simulink model "PUMAA"  (R2021a)
settings: Solver=VariableStepAuto  StartTime=0.0  StopTime=1451.7  RelTol=1e-3
undefined symbols (not defined in the file): sigbuilder_block, X, Y, Z
libraries: sm_lib x25, nesl_utility x15, pid_lib x6
settings Model: Creator=legen  LastModifiedBy=MSI

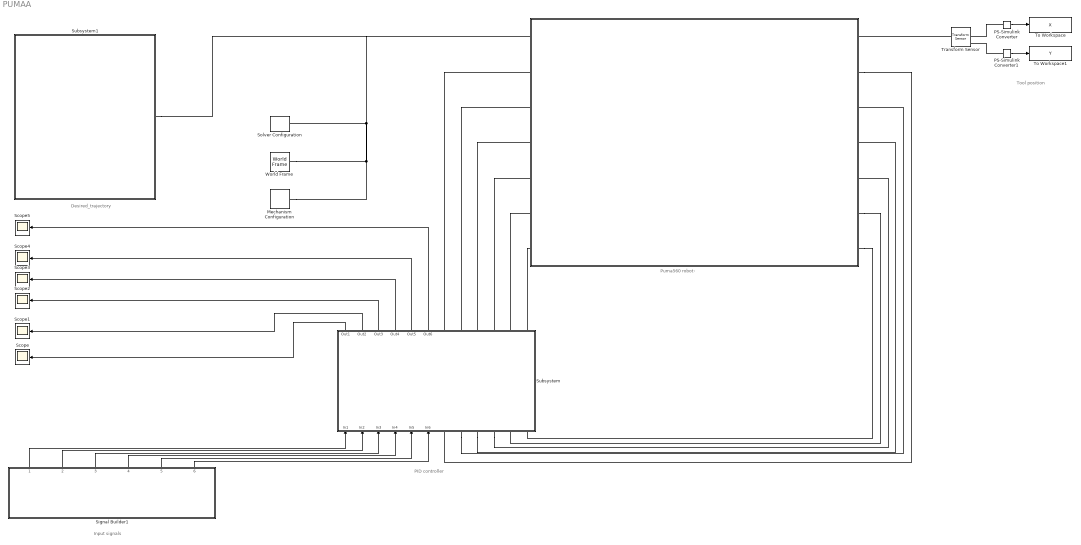
== system PUMAA ==
  note: Desired_trajectory
  note: Puma560 robot
  note: PID controller
  note: Input signals
  note: Tool position
  " ." : Subsystem
      mask Display: image('Puma.png'); % Use "Edit Image" on toolstrip to change.
  Mechanism Configuration : sm_lib/Utilities/Mechanism Configuration  UniformGravity=Constant  GravityVector=[0 0 -9.80665]  GravityVectorUnits=m/s^2  GravityUnits=m/s^2  LinearizationDelta=0.0001  JointModeTransitionNonlinearIterations=2
  PS-Simulink Converter : nesl_utility/PS-Simulink Converter  PhysicalDomain=network_engine_domain  SubClassName=ps_output  LeftPortType=input  RightPortType=output  PseudoPeriodic=off  Frequencies=[]  Unit=inherit  AffineConversion=off
      settings: SourceProductBaseCode=PW,SS
  PS-Simulink Converter1 : nesl_utility/PS-Simulink Converter  PhysicalDomain=network_engine_domain  SubClassName=ps_output  LeftPortType=input  RightPortType=output  PseudoPeriodic=off  Frequencies=[]  Unit=inherit  AffineConversion=off
      settings: SourceProductBaseCode=PW,SS
  Scope{,1..5} (6 alike) : Scope
  Signal Builder1 : Subsystem  Tag=STV Subsys  LoadFcn=sigbuilder_block('load');  StartFcn=sigbuilder_block('start');  StopFcn=sigbuilder_block('stop');  ClipboardFcn=sigbuilder_block('clipboard');  mask(Sigbuilder block){tuvar=[0:10]}
      mask help: Simulink:masks:SigbuilderBlock_MD
      mask init:
      | if ~strcmp(get_param(bdroot(gcbh),'SimulationStatus'),'stopped') tuvar = sigbuilder_block('maskInit'); end
      settings: CopyFcn=sigbuilder_block('copy');  DeleteFcn=sigbuilder_block('delete');  ModelCloseFcn=sigbuilder_block('modelClose');  PreSaveFcn=sigbuilder_block('preSave');  PauseFcn=sigbuilder_block('pause');  ContinueFcn=sigbuilder_block('continue');  NameChangeFcn=sigbuilder_block('namechange');  OpenFcn=sigbuilder_block('open',[437.6 153 550.4 359.25 ]);  CloseFcn=sigbuilder_block('close');
      mask Display: plot(0, 0, 100, 100,[2, 2, 32, 32, 2], [68, 8, 8, 68, 68],[32, 2], [38, 38], [32, 19, 2],[53, 60, 44], [32, 17, 17, 2],[16, 16, 31, 31]);txt = getActiveGroup(gcbh);text(2, 100, txt,'verticalAlignment', 'top');
  Solver Configuration : nesl_utility/Solver Configuration  PhysicalDomain=network_engine_domain  SubClassName=solver  LeftPortType=input  RightPortType=generic  Tones=[]  Harmonics=[]  SimulateNoise=off  Profile=off  UseLocalSampling=off  EnableSwitchedLinearOptims=on  FrequencyDomain=off  UseCCode=off  RelTol=0.001  AbsTol=1e-06  MinStep=1e-09  ToWorkspace=off  RevertToSquareIcSolve=off  NumHomotopyIterations=100  PhasorMode=off  PhasorModeNumHarmonics=1  DoDC=off  ResidualTolerance=1e-09  UseLocalSolver=off  LocalSolverChoice=NE_BACKWARD_EULER_ADVANCER  LocalSolverSampleTime=0.001  DoFixedCost=off  MaxNonlinIter=3  MaxModeIter=2  ComputeImpulses=off  ImpulseIterations=2  LinearAlgebra=Sparse  EquationFormulation=NE_TIME_EF  DelaysMemoryBudget=1024  AutomaticFiltering=on  FilteringTimeConstant=0.001  PartitionStorageMethod=AS_NEEDED  PartitionMemoryBudget=1024  PartitionMethod=FAST
      settings: SourceProductBaseCode=PW,SS
  Subsystem : Subsystem
      mask Display: image('PID-Controller-Explained.png'); % Use "Edit Image" on toolstrip to change.
  Subsystem1 : Subsystem
      mask Display: image('trajectory.png'); % Use "Edit Image" on toolstrip to change.
  To Workspace : ToWorkspace  VariableName=X  SampleTime=0.1
  To Workspace1 : ToWorkspace  VariableName=Y  SampleTime=0.1
  Transform Sensor : sm_lib/Frames and Transforms/Transform Sensor  MeasurementFrame=World  SenseAngle=off  SenseAxis=off  SenseAngle1=off  SenseAngle2=off  SenseAngle3=off  SenseQ=off  SenseR=off  SenseOmegaX=off  SenseOmegaY=off  SenseOmegaZ=off  SenseOmega1=off  SenseOmega2=off  SenseOmega3=off  SenseQDot=off  SenseRDot=off  SenseAlphaX=off  SenseAlphaY=off  SenseAlphaZ=off  SenseAlpha1=off  SenseAlpha2=off  SenseAlpha3=off  SenseQDDot=off  SenseRDDot=off  SenseX=on  SenseY=on  SenseZ=off  SenseRad=off  SenseAzim=off  SenseDist=off  SenseInc=off  SenseXDot=off  SenseYDot=off  SenseZDot=off  SenseRadDot=off  SenseAzimDot=off  SenseDistDot=off  SenseIncDot=off  SenseXDDot=off  SenseYDDot=off  SenseZDDot=off  SenseRadDDot=off  SenseAzimDDot=off  SenseDistDDot=off  SenseIncDDot=off
  World Frame : sm_lib/Frames and Transforms/World Frame
  wires:
  PS-Simulink Converter/1 -> To Workspace/1
  PS-Simulink Converter1/1 -> To Workspace1/1
  Signal Builder1/1(Imported_Signal 1) -> Subsystem/1(In1)
  Signal Builder1/2(Imported_Signal 2) -> Subsystem/2(In2)
  Signal Builder1/3(Imported_Signal 3) -> Subsystem/3(In3)
  Signal Builder1/4(Imported_Signal 4) -> Subsystem/4(In4)
  Signal Builder1/5(Imported_Signal 5) -> Subsystem/5(In5)
  Signal Builder1/6(Imported_Signal 6) -> Subsystem/6(In6)
  Subsystem/1(Out1) -> Scope/1
  Subsystem/2(Out2) -> Scope1/1
  Subsystem/3(Out3) -> Scope2/1
  Subsystem/4(Out4) -> Scope3/1
  Subsystem/5(Out5) -> Scope4/1
  Subsystem/6(Out6) -> Scope5/1
  connections:
  Mechanism Configuration/RConn1 -- Subsystem1/LConn1 -- " ."/LConn1 -- Solver Configuration/RConn1 -- World Frame/RConn1
  PS-Simulink Converter1/LConn1 -- Transform Sensor/RConn3
  PS-Simulink Converter/LConn1 -- Transform Sensor/RConn2
  Transform Sensor/LConn1 -- " ."/RConn1
  Subsystem/RConn1 -- " ."/LConn2
  " ."/RConn2 -- Subsystem/LConn1
  Subsystem/RConn2 -- " ."/LConn3
  Subsystem/LConn2 -- " ."/RConn3
  Subsystem/RConn3 -- " ."/LConn4
  Subsystem/LConn3 -- " ."/RConn4
  Subsystem/RConn4 -- " ."/LConn5
  Subsystem/LConn4 -- " ."/RConn5
  Subsystem/RConn5 -- " ."/LConn6
  " ."/RConn6 -- Subsystem/LConn5
  Subsystem/RConn6 -- " ."/LConn7
  " ."/RConn7 -- Subsystem/LConn6

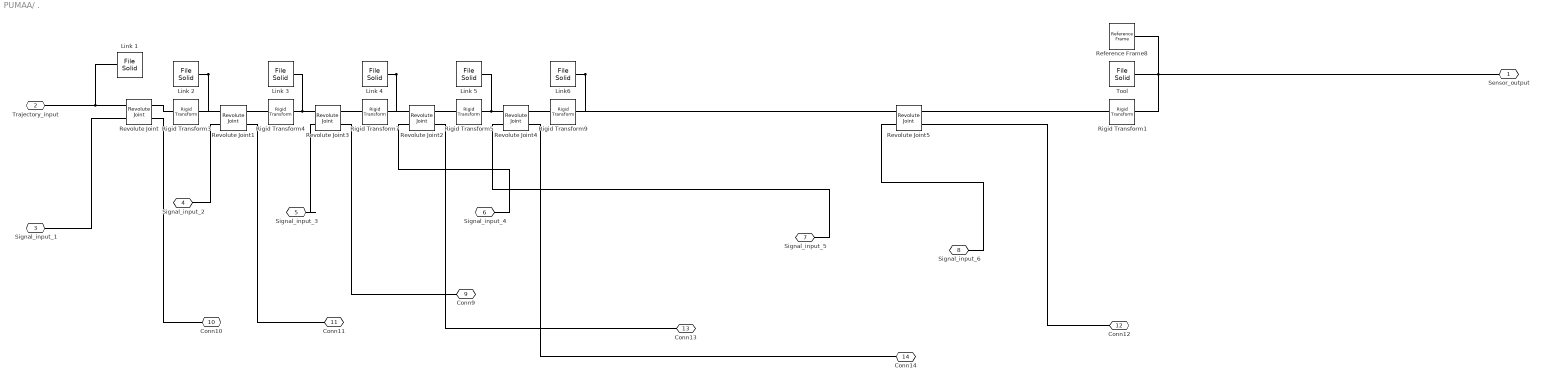
== system PUMAA/ . ==
  "Link 1 " : sm_lib/Body Elements/File Solid  ExtGeomFileName=C:\Users\MSI\Downloads\Robotics\Robotics\link0.stl  UnitType=Custom  ExtGeomFileUnits=m  StepReaderType=HEX  ExportConvexHullGeometry=off  InertiaType=Custom  Mass=0  MassUnits=kg  CenterOfMass=[0 0 0]  CenterOfMassUnits=m  MomentsOfInertia=[0 0.35 0]  MomentsOfInertiaUnits=kg*m^2  ProductsOfInertia=[0 0 0]  ProductsOfInertiaUnits=kg*m^2  BasedOnType=Mass  Density=1000  DensityUnits=kg/m^3  DoExposeReferenceFrame=on  SerializedFrames=<Frames/>  GraphicType=FromGeometry  MarkerShape=Sphere  MarkerSize=10  GraphicVisPropType=SimpleVisualProperties  GraphicDiffuseColor=[0.5 0.5 0.5]  GraphicSpecularColor=[0.5 0.5 0.5 1.0]  GraphicAmbientColor=[0.15 0.15 0.15 1.0]  GraphicEmissiveColor=[0.0 0.0 0.0 1.0]  GraphicShininess=75  GraphicOpacity=1.0
  Link 2 : sm_lib/Body Elements/File Solid  ExtGeomFileName=C:\Users\MSI\Downloads\Robotics\Robotics\link1.stl  UnitType=Custom  ExtGeomFileUnits=m  StepReaderType=HEX  ExportConvexHullGeometry=off  InertiaType=Custom  Mass=17.4  MassUnits=kg  CenterOfMass=[-0.3638 0.006 0.2275]  CenterOfMassUnits=m  MomentsOfInertia=[0.13 0.524 0.539]  MomentsOfInertiaUnits=kg*m^2  ProductsOfInertia=[0 0 0]  ProductsOfInertiaUnits=kg*m^2  BasedOnType=Density  Density=1000  DensityUnits=kg/m^3  DoExposeReferenceFrame=on  SerializedFrames=<Frames/>  GraphicType=FromGeometry  MarkerShape=Sphere  MarkerSize=10  GraphicVisPropType=SimpleVisualProperties  GraphicDiffuseColor=[0.5 0.5 0.5]  GraphicSpecularColor=[0.5 0.5 0.5 1.0]  GraphicAmbientColor=[0.15 0.15 0.15 1.0]  GraphicEmissiveColor=[0.0 0.0 0.0 1.0]  GraphicShininess=75  GraphicOpacity=1.0
  "Link 3 " : sm_lib/Body Elements/File Solid  ExtGeomFileName=C:\Users\MSI\Downloads\Robotics\Robotics\link2.stl  UnitType=Custom  ExtGeomFileUnits=m  StepReaderType=HEX  ExportConvexHullGeometry=off  InertiaType=Custom  Mass=4.8  MassUnits=kg  CenterOfMass="[-0.0203     -0.0141     0.07]"  CenterOfMassUnits=m  MomentsOfInertia=[0.066 0.086 0.0125]  MomentsOfInertiaUnits=kg*m^2  ProductsOfInertia=[0 0 0]  ProductsOfInertiaUnits=kg*m^2  BasedOnType=Density  Density=1000  DensityUnits=kg/m^3  DoExposeReferenceFrame=on  SerializedFrames=<Frames/>  GraphicType=FromGeometry  MarkerShape=Sphere  MarkerSize=10  GraphicVisPropType=SimpleVisualProperties  GraphicDiffuseColor=[0.5 0.5 0.5]  GraphicSpecularColor=[0.5 0.5 0.5 1.0]  GraphicAmbientColor=[0.15 0.15 0.15 1.0]  GraphicEmissiveColor=[0.0 0.0 0.0 1.0]  GraphicShininess=75  GraphicOpacity=1.0
  Link 4 : sm_lib/Body Elements/File Solid  ExtGeomFileName=C:\Users\MSI\Downloads\Robotics\Robotics\link3.stl  UnitType=Custom  ExtGeomFileUnits=m  StepReaderType=HEX  ExportConvexHullGeometry=off  InertiaType=Custom  Mass=0.82  MassUnits=kg  CenterOfMass="[0           0.019       0]"  CenterOfMassUnits=m  MomentsOfInertia=[0.0018 0.0013 0.0018]  MomentsOfInertiaUnits=kg*m^2  ProductsOfInertia=[0 0 0]  ProductsOfInertiaUnits=kg*m^2  BasedOnType=Density  Density=1000  DensityUnits=kg/m^3  DoExposeReferenceFrame=on  SerializedFrames=<Frames/>  GraphicType=FromGeometry  MarkerShape=Sphere  MarkerSize=10  GraphicVisPropType=SimpleVisualProperties  GraphicDiffuseColor=[0.5 0.5 0.5]  GraphicSpecularColor=[0.5 0.5 0.5 1.0]  GraphicAmbientColor=[0.15 0.15 0.15 1.0]  GraphicEmissiveColor=[0.0 0.0 0.0 1.0]  GraphicShininess=75  GraphicOpacity=1.0
  Link 5 : sm_lib/Body Elements/File Solid  ExtGeomFileName=C:\Users\MSI\Downloads\Robotics\Robotics\link4.stl  UnitType=Custom  ExtGeomFileUnits=m  StepReaderType=HEX  ExportConvexHullGeometry=off  InertiaType=Custom  Mass=0.34  MassUnits=kg  CenterOfMass=[0 0 0]  CenterOfMassUnits=m  MomentsOfInertia=[0.0003 0.0004 0.0003]  MomentsOfInertiaUnits=kg*m^2  ProductsOfInertia=[0 0 0]  ProductsOfInertiaUnits=kg*m^2  BasedOnType=Density  Density=1000  DensityUnits=kg/m^3  DoExposeReferenceFrame=on  SerializedFrames=<Frames/>  GraphicType=FromGeometry  MarkerShape=Sphere  MarkerSize=10  GraphicVisPropType=SimpleVisualProperties  GraphicDiffuseColor=[0.5 0.5 0.5]  GraphicSpecularColor=[0.5 0.5 0.5 1.0]  GraphicAmbientColor=[0.15 0.15 0.15 1.0]  GraphicEmissiveColor=[0.0 0.0 0.0 1.0]  GraphicShininess=75  GraphicOpacity=1.0
  Link6 : sm_lib/Body Elements/File Solid  ExtGeomFileName=C:\Users\MSI\Downloads\Robotics\Robotics\link5.stl  UnitType=Custom  ExtGeomFileUnits=m  StepReaderType=HEX  ExportConvexHullGeometry=off  InertiaType=Custom  Mass=0.09  MassUnits=kg  CenterOfMass=[0 0 0.032]  CenterOfMassUnits=m  MomentsOfInertia=[0.00015 0.00015 4e-5]  MomentsOfInertiaUnits=kg*m^2  ProductsOfInertia=[0 0 0]  ProductsOfInertiaUnits=kg*m^2  BasedOnType=Density  Density=1000  DensityUnits=kg/m^3  DoExposeReferenceFrame=on  SerializedFrames=<Frames/>  GraphicType=FromGeometry  MarkerShape=Sphere  MarkerSize=10  GraphicVisPropType=SimpleVisualProperties  GraphicDiffuseColor=[0.5 0.5 0.5]  GraphicSpecularColor=[0.5 0.5 0.5 1.0]  GraphicAmbientColor=[0.15 0.15 0.15 1.0]  GraphicEmissiveColor=[0.0 0.0 0.0 1.0]  GraphicShininess=75  GraphicOpacity=1.0
  Reference Frame8 : sm_lib/Frames and Transforms/Reference Frame
  Revolute Joint{,1..5} (6 alike) : sm_lib/Joints/Revolute Joint  JointMode=Normal  SenseConstraintForce=off  SenseConstraintForceX=off  SenseConstraintForceY=off  SenseConstraintForceZ=off  SenseConstraintTorque=off  SenseConstraintTorqueX=off  SenseConstraintTorqueY=off  SenseConstraintTorqueZ=off  SenseTotalForce=off  SenseTotalForceX=off  SenseTotalForceY=off  SenseTotalForceZ=off  SenseTotalTorque=off  SenseTotalTorqueX=off  SenseTotalTorqueY=off  SenseTotalTorqueZ=off  CompositeWrenchDir=FollowerOnBase  CompositeWrenchFrame=BaseFrame  EquilibriumPosition=0  EquilibriumPositionUnits=deg  SpringStiffness=0  SpringStiffnessUnits=N*m/deg  DampingCoefficient=0  DampingCoefficientUnits=N*m/(deg/s)  TorqueActuationMode=ComputedTorque  MotionActuationMode=InputMotion  SensePosition=on  SenseVelocity=off  SenseAcceleration=off  SenseTorqueForce=off  SenseLowerLimitTorqueForce=off  SenseUpperLimitTorqueForce=off  LowerLimitSpecify=off  LowerLimitBound=-90  LowerLimitBoundUnits=deg  LowerLimitStiffness=1e4  LowerLimitStiffnessUnits=N*m/deg  LowerLimitDamping=10  LowerLimitDampingUnits=N*m/(deg/s)  LowerLimitTransitionRegionWidth=0.1  LowerLimitTransitionRegionWidthUnits=deg  UpperLimitSpecify=off  UpperLimitBound=90  UpperLimitBoundUnits=deg  UpperLimitStiffness=1e4  UpperLimitStiffnessUnits=N*m/deg  UpperLimitDamping=10  UpperLimitDampingUnits=N*m/(deg/s)  UpperLimitTransitionRegionWidth=0.1  UpperLimitTransitionRegionWidthUnits=deg  PositionTargetSpecify=off  PositionTargetPriority=High  PositionTargetValue=0  PositionTargetValueUnits=deg  VelocityTargetSpecify=off  VelocityTargetPriority=High  VelocityTargetValue=0  VelocityTargetValueUnits=deg/s
  Rigid Transform1 : sm_lib/Frames and Transforms/Rigid Transform  TranslationMethod=Cartesian  TranslationStandardOffset=0  TranslationLengthUnit=m  TranslationStandardAxis=+Z  TranslationCartesianOffset=[-0.037 -0.04 0.045]  TranslationROffset=0  TranslationROffsetUnits=m  TranslationZOffset=0  TranslationZOffsetUnits=m  TranslationThetaOffset=0  TranslationThetaOffsetUnits=deg  RotationMethod=ArbitraryAxis  RotationAngleUnits=rad  RotationStandardAxis=-X  RotationAngle=0  RotationArbitraryAxis=[0 0 1]  FollAlignAxisA=-Y  BaseAlignAxisA=+Z  FollAlignAxisB=+X  BaseAlignAxisB=+X  RotationSequenceAxes=FollowerAxes  RotationSequence=XYX  RotationSequenceAngles=[0 0 0]  RotationSequenceAnglesUnits=deg  RotationMatrix=[1 0 0; 0 0 1; 0 -1 0]
  Rigid Transform3 : sm_lib/Frames and Transforms/Rigid Transform  TranslationMethod=None  TranslationStandardOffset=0  TranslationLengthUnit=m  TranslationStandardAxis=+Z  TranslationCartesianOffset=[0.5 0 0]  TranslationROffset=0  TranslationROffsetUnits=m  TranslationZOffset=0  TranslationZOffsetUnits=m  TranslationThetaOffset=0  TranslationThetaOffsetUnits=deg  RotationMethod=RotationMatrix  RotationAngleUnits=rad  RotationStandardAxis=-X  RotationAngle=pi/2  RotationArbitraryAxis=[0 0 1]  FollAlignAxisA=+X  BaseAlignAxisA=+X  FollAlignAxisB=+Y  BaseAlignAxisB=+Z  RotationSequenceAxes=FollowerAxes  RotationSequence=XYX  RotationSequenceAngles=[0 0 0]  RotationSequenceAnglesUnits=deg  RotationMatrix=[1 0 0; 0 0 -1; 0 1 0]
  Rigid Transform4 : sm_lib/Frames and Transforms/Rigid Transform  TranslationMethod=Cartesian  TranslationStandardOffset=0  TranslationLengthUnit=m  TranslationStandardAxis=+Z  TranslationCartesianOffset=[0.4318 0 0]  TranslationROffset=0  TranslationROffsetUnits=m  TranslationZOffset=0  TranslationZOffsetUnits=m  TranslationThetaOffset=0  TranslationThetaOffsetUnits=deg  RotationMethod=None  RotationAngleUnits=rad  RotationStandardAxis=+Y  RotationAngle=pi/2  RotationArbitraryAxis=[0 0 1]  FollAlignAxisA=+Z  BaseAlignAxisA=+Z  FollAlignAxisB=+X  BaseAlignAxisB=+X  RotationSequenceAxes=FollowerAxes  RotationSequence=XYX  RotationSequenceAngles=[0 0 0]  RotationSequenceAnglesUnits=deg  RotationMatrix=[1 0 0; 0 1 0; 0 0 1]
  Rigid Transform5 : sm_lib/Frames and Transforms/Rigid Transform  TranslationMethod=Cartesian  TranslationStandardOffset=0  TranslationLengthUnit=m  TranslationStandardAxis=+Z  TranslationCartesianOffset=[0 0 0.4318]  TranslationROffset=0  TranslationROffsetUnits=m  TranslationZOffset=0  TranslationZOffsetUnits=m  TranslationThetaOffset=0  TranslationThetaOffsetUnits=deg  RotationMethod=RotationMatrix  RotationAngleUnits=rad  RotationStandardAxis=-X  RotationAngle=pi/2  RotationArbitraryAxis=[0 0 1]  FollAlignAxisA=-Y  BaseAlignAxisA=+Z  FollAlignAxisB=+X  BaseAlignAxisB=+Y  RotationSequenceAxes=FollowerAxes  RotationSequence=XYX  RotationSequenceAngles=[0 0 0]  RotationSequenceAnglesUnits=deg  RotationMatrix=[1 0 0; 0 0 -1; 0 1 0]
  Rigid Transform7 : sm_lib/Frames and Transforms/Rigid Transform  TranslationMethod=Cartesian  TranslationStandardOffset=0  TranslationLengthUnit=m  TranslationStandardAxis=+Z  TranslationCartesianOffset=[0.0203 0 0.15005 ]  TranslationROffset=0  TranslationROffsetUnits=m  TranslationZOffset=0  TranslationZOffsetUnits=m  TranslationThetaOffset=0  TranslationThetaOffsetUnits=deg  RotationMethod=RotationMatrix  RotationAngleUnits=rad  RotationStandardAxis=+Y  RotationAngle=pi/2  RotationArbitraryAxis=[0 0 1]  FollAlignAxisA=+X  BaseAlignAxisA=-Z  FollAlignAxisB=+Y  BaseAlignAxisB=-Y  RotationSequenceAxes=FollowerAxes  RotationSequence=XYX  RotationSequenceAngles=[0 0 0]  RotationSequenceAnglesUnits=deg  RotationMatrix=[1 0 0; 0 0 1; 0 -1 0]
  Rigid Transform9 : sm_lib/Frames and Transforms/Rigid Transform  TranslationMethod=None  TranslationStandardOffset=0  TranslationLengthUnit=m  TranslationStandardAxis=+Z  TranslationCartesianOffset=[0 -0.2 0]  TranslationROffset=0  TranslationROffsetUnits=m  TranslationZOffset=0  TranslationZOffsetUnits=m  TranslationThetaOffset=0  TranslationThetaOffsetUnits=deg  RotationMethod=RotationMatrix  RotationAngleUnits=rad  RotationStandardAxis=-X  RotationAngle=pi/2  RotationArbitraryAxis=[0 0 1]  FollAlignAxisA=+X  BaseAlignAxisA=+Z  FollAlignAxisB=+Z  BaseAlignAxisB=-Y  RotationSequenceAxes=FollowerAxes  RotationSequence=XYX  RotationSequenceAngles=[0 0 0]  RotationSequenceAnglesUnits=deg  RotationMatrix=[1 0 0; 0 0 1; 0 -1 0]
  Tool : sm_lib/Body Elements/File Solid  ExtGeomFileName=C:\Users\MSI\Downloads\Robotics\Robotics\Binzel Segment Holder Abirob A300 ECO.STL  UnitType=Custom  ExtGeomFileUnits=mm  StepReaderType=HEX  ExportConvexHullGeometry=off  InertiaType=CalculateFromGeometry  Mass=1  MassUnits=kg  CenterOfMass=[0 0 0]  CenterOfMassUnits=m  MomentsOfInertia=[1 1 1]  MomentsOfInertiaUnits=kg*m^2  ProductsOfInertia=[0 0 0]  ProductsOfInertiaUnits=kg*m^2  BasedOnType=Density  Density=1000  DensityUnits=kg/m^3  DoExposeReferenceFrame=on  SerializedFrames=<Frames/>  GraphicType=FromGeometry  MarkerShape=Sphere  MarkerSize=10  GraphicVisPropType=SimpleVisualProperties  GraphicDiffuseColor=[1.0 0.0 0.2]  GraphicSpecularColor=[0.5 0.5 0.5 1.0]  GraphicAmbientColor=[0.15 0.15 0.15 1.0]  GraphicEmissiveColor=[0.0 0.0 0.0 1.0]  GraphicShininess=75  GraphicOpacity=1.0
  Sensor_output : PMIOPort  Side=Right
  Trajectory_input : PMIOPort  Port=2  Side=Left
  Signal_input_1 : PMIOPort  Port=3  Side=Left
  Signal_input_2 : PMIOPort  Port=4  Side=Left
  Signal_input_3 : PMIOPort  Port=5  Side=Left
  Signal_input_4 : PMIOPort  Port=6  Side=Left
  Signal_input_5 : PMIOPort  Port=7  Side=Left
  Signal_input_6 : PMIOPort  Port=8  Side=Left
  Conn9 : PMIOPort  Port=9  Side=Right
  Conn10 : PMIOPort  Port=10  Side=Right
  Conn11 : PMIOPort  Port=11  Side=Right
  Conn12 : PMIOPort  Port=12  Side=Right
  Conn13 : PMIOPort  Port=13  Side=Right
  Conn14 : PMIOPort  Port=14  Side=Right
  connections:
  Link6/RConn1 -- Rigid Transform9/RConn1 -- Revolute Joint5/LConn1
  Rigid Transform1/RConn1 -- Sensor_output/RConn1 -- Reference Frame8/RConn1 -- Tool/RConn1
  Rigid Transform4/LConn1 -- Revolute Joint1/RConn1
  Rigid Transform7/LConn1 -- Revolute Joint3/RConn1
  Signal_input_5/RConn1 -- Revolute Joint4/LConn2
  Revolute Joint5/RConn1 -- Rigid Transform1/LConn1
  Revolute Joint/LConn1 -- Trajectory_input/RConn1 -- "Link 1 "/RConn1
  Link 2/RConn1 -- Rigid Transform3/RConn1 -- Revolute Joint1/LConn1
  Revolute Joint4/RConn2 -- Conn14/RConn1
  Rigid Transform5/RConn1 -- Link 5/RConn1 -- Revolute Joint4/LConn1
  Conn11/RConn1 -- Revolute Joint1/RConn2
  Rigid Transform4/RConn1 -- "Link 3 "/RConn1 -- Revolute Joint3/LConn1
  Revolute Joint2/RConn2 -- Conn13/RConn1
  Revolute Joint/RConn1 -- Rigid Transform3/LConn1
  Rigid Transform9/LConn1 -- Revolute Joint4/RConn1
  Rigid Transform5/LConn1 -- Revolute Joint2/RConn1
  Link 4/RConn1 -- Rigid Transform7/RConn1 -- Revolute Joint2/LConn1
  Conn10/RConn1 -- Revolute Joint/RConn2
  Signal_input_4/RConn1 -- Revolute Joint2/LConn2
  Revolute Joint3/RConn2 -- Conn9/RConn1
  Conn12/RConn1 -- Revolute Joint5/RConn2
  Signal_input_6/RConn1 -- Revolute Joint5/LConn2
  Signal_input_3/RConn1 -- Revolute Joint3/LConn2
  Signal_input_2/RConn1 -- Revolute Joint1/LConn2
  Revolute Joint/LConn2 -- Signal_input_1/RConn1

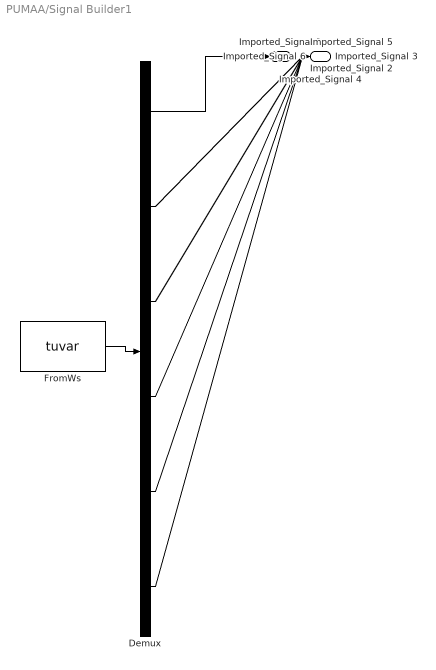
== system PUMAA/Signal Builder1 ==
  Demux : Demux  Tag=STV Demux  Outputs=6
      settings: DisplayOption=none
  FromWs : FromWorkspace  Tag=STV FromWs  VariableName=tuvar
      SigBuilderData=|
      | common.afterFinalStr = 'Extrapolate'
      | common.sampleTime = 0
      | dataSet.timeRange = [0.1 1451.8]
      | dataSet.name = 'Imported_Group 1'
      | sbobj.Name = 'Signal Builder'
      | sbobj.Groups.Name = 'Imported_Group 1'
      | sbobj.Groups.Signals(1).Name = 'Imported_Signal 1'
      | sbobj.Groups.Signals(1).XData = [0.1 0.2 0.3 0.4 0.5 0.6 0.7 0.8 0.9 1 1.1 1.2 ... (14518 elements, 1x14518)]
      | sbobj.Groups.Signals(1).YData = [2.13521 2.13543 2.1355 2.13558 2.13566 2.13574 2.13581 2.13589 2.13597 2.13605 2.13613 2.1362 ... (14518 elements, 1x14518)]
      | sbobj.Groups.Signals(2).Name = 'Imported_Signal 2'
      | sbobj.Groups.Signals(2).XData = [0.1 0.2 0.3 0.4 0.5 0.6 0.7 0.8 0.9 1 1.1 1.2 ... (14518 elements, 1x14518)]
      | sbobj.Groups.Signals(2).YData = [2.38325 2.38326 2.38347 2.38367 2.38388 2.38408 2.38429 2.38449 2.3847 2.3849 2.38511 2.38531 ... (14518 elements, 1x14518)]
      | sbobj.Groups.Signals(3).Name = 'Imported_Signal 3'
      | sbobj.Groups.Signals(3).XData = [0.1 0.2 0.3 0.4 0.5 0.6 0.7 0.8 0.9 1 1.1 1.2 ... (14518 elements, 1x14518)]
      | sbobj.Groups.Signals(3).YData = [-0.00816894 -0.00820264 -0.00861319 -0.00902339 -0.00943325 -0.00984276 -0.0102519 -0.0106607 -0.0110692 -0.0114773 -0.0118851 -0.0122925 ... (14518 elements, 1x14518)]
      | sbobj.Groups.Signals(4).Name = 'Imported_Signal 4'
      | sbobj.Groups.Signals(4).XData = [0.1 0.2 0.3 0.4 0.5 0.6 0.7 0.8 0.9 1 1.1 1.2 ... (14518 elements, 1x14518)]
      | sbobj.Groups.Signals(4).YData = [-1.51868e-16 -1.51864e-16 -1.51819e-16 -1.51774e-16 -1.5173e-16 -1.51685e-16 -1.5164e-16 -1.51596e-16 -1.51551e-16 -1.51507e-16 -1.51462e-16 -1.51418e-16 ... (14518 elements, 1x14518)]
      | sbobj.Groups.Signals(5).Name = 'Imported_Signal 5'
      | sbobj.Groups.Signals(5).XData = [0.1 0.2 0.3 0.4 0.5 0.6 0.7 0.8 0.9 1 1.1 1.2 ... (14518 elements, 1x14518)]
      | sbobj.Groups.Signals(5).YData = [0.766516 0.766533 0.766738 0.766943 0.767147 0.767352 0.767556 0.767761 0.767965 0.768168 0.768372 0.768576 ... (14518 elements, 1x14518)]
      | sbobj.Groups.Signals(6).Name = 'Imported_Signal 6'
      | sbobj.Groups.Signals(6).XData = [0.1 0.2 0.3 0.4 0.5 0.6 0.7 0.8 0.9 1 1.1 1.2 ... (14518 elements, 1x14518)]
      | sbobj.Groups.Signals(6).YData = [0 0 0 0 0 0 0 0 0 0 0 0 ... (14518 elements, 1x14518)]
      | sbobj.Groups.TimeRange = [0.1 325.6]
  Imported_Signal 1 : Outport  Tag=STV Outport
  Imported_Signal 2 : Outport  Tag=STV Outport  Port=2
  Imported_Signal 3 : Outport  Tag=STV Outport  Port=3
  Imported_Signal 4 : Outport  Tag=STV Outport  Port=4
  Imported_Signal 5 : Outport  Tag=STV Outport  Port=5
  Imported_Signal 6 : Outport  Tag=STV Outport  Port=6
  wires:
  Demux/1 -> Imported_Signal 1/1
  FromWs/1 -> Demux/1
  Demux/2 -> Imported_Signal 2/1
  Demux/3 -> Imported_Signal 3/1
  Demux/4 -> Imported_Signal 4/1
  Demux/5 -> Imported_Signal 5/1
  Demux/6 -> Imported_Signal 6/1

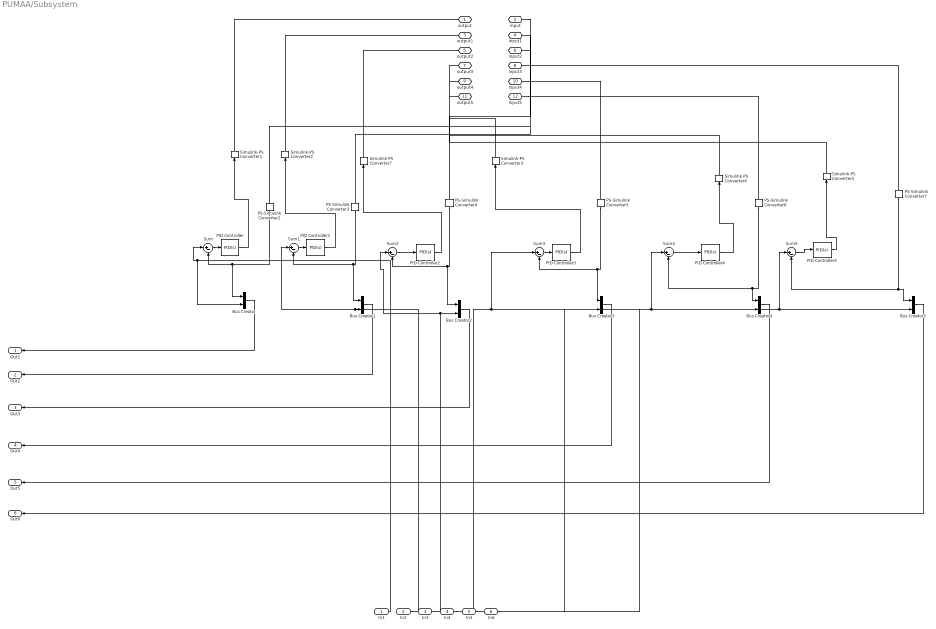
== system PUMAA/Subsystem ==
  In1 : Inport
  In2 : Inport  Port=2
  In3 : Inport  Port=3
  In4 : Inport  Port=4
  In5 : Inport  Port=5
  In6 : Inport  Port=6
  Bus Creator{,1..5} (6 alike) : BusCreator  Inputs=2
  PID Controller{,1..5} (6 alike) : pid_lib/PID Controller  Controller=PID  Form=Parallel  TimeDomain=Continuous-time  UseExternalTs=off  SampleTime=-1  IntegratorMethod=Forward Euler  FilterMethod=Forward Euler  ControllerParametersSource=internal  P=1  I=1  D=0  UseFilter=on  N=100  TunerSelectOption=Frequency Response Based  InitialConditionSource=internal  InitialConditionForIntegrator=0  InitialConditionForFilter=0  DifferentiatorICPrevScaledInput=0  ExternalReset=none  TrackingMode=off  Kt=1  LimitOutput=off  SatLimitsSource=internal  UpperSaturationLimit=inf  LowerSaturationLimit=-inf  LinearizeAsGain=on  AntiWindupMode=none  Kb=1  POutMin=[]  POutMax=[]  IOutMin=[]  IOutMax=[]  DOutMin=[]  DOutMax=[]  NOutMin=[]  NOutMax=[]  SumOutMin=[]  SumOutMax=[]  SaturationOutMin=[]  SaturationOutMax=[]  PParamMin=[]  PParamMax=[]  IParamMin=[]  IParamMax=[]  DParamMin=[]  DParamMax=[]  NParamMin=[]  NParamMax=[]  KbParamMin=[]  KbParamMax=[]  KtParamMin=[]  KtParamMax=[]  KbOutMin=[]  KbOutMax=[]  KtOutMin=[]  KtOutMax=[]  IntegratorOutMin=[]  IntegratorOutMax=[]  FilterOutMin=[]  FilterOutMax=[]  SumI1OutMin=[]  SumI1OutMax=[]  SumI2OutMin=[]  SumI2OutMax=[]  SumI3OutMin=[]  SumI3OutMax=[]  SumI4OutMin=[]  SumI4OutMax=[]  SumDOutMin=[]  SumDOutMax=[]  DifferentiatorOutMin=[]  DifferentiatorOutMax=[]  FilterDiffOutCoefMin=[]  FilterDiffOutCoefMax=[]  ReciprocalOutMin=[]  ReciprocalOutMax=[]  SumDenOutMin=[]  SumDenOutMax=[]  SumNumOutMin=[]  SumNumOutMax=[]  DivideOutMin=[]  DivideOutMax=[]  UdiffTsProdOutMin=[]  UdiffTsProdOutMax=[]  NTsProdOutMin=[]  NTsProdOutMax=[]  UintegralTsProdOutMin=[]  UintegralTsProdOutMax=[]  UngainTsProdOutMin=[]  UngainTsProdOutMax=[]  IntegratorContinuousStateAttributes=''  IntegratorStateMustResolveToSignalObject=off  IntegratorRTWStateStorageClass=Auto  FilterContinuousStateAttributes=''  FilterStateMustResolveToSignalObject=off  FilterRTWStateStorageClass=Auto  ParallelPVariant=InternalParameters  IdealPVariant=Disabled  IVariant=InternalParameters  DVariant=InternalParameters  IntegratorVariant=Continuous  SatVariant=Disabled  AWVariant=Passthrough  PCopyVariant=Disabled  TRVariant=Disabled  FdbkBlocksVariant=Forward  IdealPFdbkVariant=Disabled  SatFdbkVariant=Disabled  DerivativeFilterVariant=ContFilter  NVariant=InternalParameters  NCopyVariant=Disabled  FilterICVariant=InternalICsFilter  IntegratorICVariant=InternalICs  ExternalResetVariant=Disabled  TRSumVariant=Passthrough  SumFdbkVariant=Disabled  SumVariant=Sum_PID  TsampFilterVariant=InternalTs  TsampNgainVariant=Passthrough  TsampIntegralVariant=Passthrough  ExternalSaturationOutDataTypeStr=Inherit: Same as second input
  PS-Simulink Converter{2..7} (6 alike) : nesl_utility/PS-Simulink Converter  PhysicalDomain=network_engine_domain  SubClassName=ps_output  LeftPortType=input  RightPortType=output  PseudoPeriodic=off  Frequencies=[]  Unit=inherit  AffineConversion=off
      settings: SourceProductBaseCode=PW,SS
  Simulink-PS Converter{1..5,7} (6 alike) : nesl_utility/Simulink-PS Converter  PhysicalDomain=network_engine_domain  SubClassName=ps_input  LeftPortType=input  RightPortType=output  PseudoPeriodic=off  Frequencies=[]  NoiseDistribution=none  NoiseParameters=[]  Unit=1  AffineConversion=off  FilteringAndDerivatives=filter  SimscapeFilterOrder=2  InputFilterTimeConstant=0.001  UdotUserProvided=0
      settings: SourceProductBaseCode=PW,SS
  Sum{,1..5} (6 alike) : Sum  Inputs=|+-
  output : PMIOPort  Side=Right
  input : PMIOPort  Port=2  Side=Left
  output1 : PMIOPort  Port=3  Side=Right
  input1 : PMIOPort  Port=4  Side=Left
  output2 : PMIOPort  Port=5  Side=Right
  input2 : PMIOPort  Port=6  Side=Left
  output3 : PMIOPort  Port=7  Side=Right
  input3 : PMIOPort  Port=8  Side=Left
  output4 : PMIOPort  Port=9  Side=Right
  input4 : PMIOPort  Port=10  Side=Left
  output5 : PMIOPort  Port=11  Side=Right
  input5 : PMIOPort  Port=12  Side=Left
  Out1 : Outport
  Out2 : Outport  Port=2
  Out3 : Outport  Port=3
  Out4 : Outport  Port=4
  Out5 : Outport  Port=5
  Out6 : Outport  Port=6
  wires:
  Bus Creator1/1 -> Out2/1
  Sum5/1 -> PID Controller5/1
  In4/1 -> Sum3/1, Bus Creator3/2
  In2/1 -> Sum1/1, Bus Creator1/2
  Sum1/1 -> PID Controller1/1
  PS-Simulink Converter7/1 -> Bus Creator5/1, Sum5/2
  In5/1 -> Bus Creator4/2, Sum4/1
  PID Controller3/1 -> Simulink-PS Converter3/1
  PS-Simulink Converter2/1 -> Sum/2, Bus Creator/1
  PS-Simulink Converter3/1 -> Sum1/2, Bus Creator1/1
  PID Controller/1 -> Simulink-PS Converter1/1
  Sum/1 -> PID Controller/1
  In6/1 -> Bus Creator5/2, Sum5/1
  PID Controller1/1 -> Simulink-PS Converter2/1
  PS-Simulink Converter6/1 -> Sum4/2, Bus Creator4/1
  PS-Simulink Converter4/1 -> Bus Creator2/1, Sum2/2
  Bus Creator3/1 -> Out4/1
  Sum2/1 -> PID Controller2/1
  PID Controller2/1 -> Simulink-PS Converter7/1
  PID Controller5/1 -> Simulink-PS Converter5/1
  Sum4/1 -> PID Controller4/1
  PS-Simulink Converter5/1 -> Sum3/2, Bus Creator3/1
  In3/1 -> Sum2/1, Bus Creator2/2
  Bus Creator4/1 -> Out5/1
  Bus Creator2/1 -> Out3/1
  PID Controller4/1 -> Simulink-PS Converter4/1
  Bus Creator5/1 -> Out6/1
  Sum3/1 -> PID Controller3/1
  Bus Creator/1 -> Out1/1
  In1/1 -> Bus Creator/2, Sum/1
  connections:
  Simulink-PS Converter5/RConn1 -- output5/RConn1
  input5/RConn1 -- PS-Simulink Converter6/LConn1
  PS-Simulink Converter2/LConn1 -- input1/RConn1
  Simulink-PS Converter2/RConn1 -- output1/RConn1
  input/RConn1 -- PS-Simulink Converter4/LConn1
  Simulink-PS Converter4/RConn1 -- output4/RConn1
  Simulink-PS Converter3/RConn1 -- output3/RConn1
  PS-Simulink Converter7/LConn1 -- input3/RConn1
  Simulink-PS Converter7/RConn1 -- output2/RConn1
  Simulink-PS Converter1/RConn1 -- output/RConn1
  PS-Simulink Converter3/LConn1 -- input2/RConn1
  input4/RConn1 -- PS-Simulink Converter5/LConn1

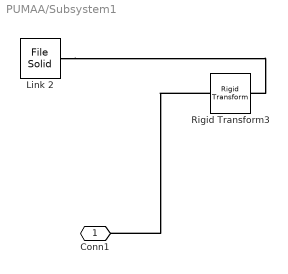
== system PUMAA/Subsystem1 ==
  Link 2 : sm_lib/Body Elements/File Solid  ExtGeomFileName=C:\Users\MSI\Downloads\Robotics\Robotics\trajectory.STL  UnitType=Custom  ExtGeomFileUnits=mm  StepReaderType=HEX  ExportConvexHullGeometry=off  InertiaType=Custom  Mass=17.4  MassUnits=kg  CenterOfMass=[-0.3638 0.006 0.2275]  CenterOfMassUnits=m  MomentsOfInertia=[0.13 0.524 0.539]  MomentsOfInertiaUnits=kg*m^2  ProductsOfInertia=[0 0 0]  ProductsOfInertiaUnits=kg*m^2  BasedOnType=Density  Density=1000  DensityUnits=kg/m^3  DoExposeReferenceFrame=on  SerializedFrames=<Frames/>  GraphicType=FromGeometry  MarkerShape=Sphere  MarkerSize=10  GraphicVisPropType=SimpleVisualProperties  GraphicDiffuseColor=[0.0 0.8 0.8]  GraphicSpecularColor=[0.5 0.5 0.5 1.0]  GraphicAmbientColor=[0.15 0.15 0.15 1.0]  GraphicEmissiveColor=[0.0 0.0 0.0 1.0]  GraphicShininess=75  GraphicOpacity=1.0
  Rigid Transform3 : sm_lib/Frames and Transforms/Rigid Transform  TranslationMethod=Cartesian  TranslationStandardOffset=0  TranslationLengthUnit=m  TranslationStandardAxis=+Z  TranslationCartesianOffset=[0.24 -0.5 -0.5]  TranslationROffset=0  TranslationROffsetUnits=m  TranslationZOffset=0  TranslationZOffsetUnits=m  TranslationThetaOffset=0  TranslationThetaOffsetUnits=deg  RotationMethod=None  RotationAngleUnits=rad  RotationStandardAxis=-X  RotationAngle=pi/2  RotationArbitraryAxis=[0 0 1]  FollAlignAxisA=+X  BaseAlignAxisA=+X  FollAlignAxisB=+Y  BaseAlignAxisB=+Z  RotationSequenceAxes=FollowerAxes  RotationSequence=XYX  RotationSequenceAngles=[0 0 0]  RotationSequenceAnglesUnits=deg  RotationMatrix=[1 0 0; 0 0 -1; 0 1 0]
  Conn1 : PMIOPort  Side=Left
  connections:
  Rigid Transform3/LConn1 -- Conn1/RConn1
  Link 2/RConn1 -- Rigid Transform3/RConn1
